simulink model "simple_simulation"  (R2025b)
settings: Solver=ode45  StartTime=0.0  StopTime=30  RelTol=1e-3
values from neighbouring files (symbols this model uses):
  M = SX.zeros(n, n)    [get_wheeled_robot_model.m]    (also in simple_model.m = 19)
  m_w = 1.0    (= 1)    [get_wheeled_robot_model.m]    (also in simple_model.m)
  N = 40    [simple_ocp.m]    (also in solver_ocp.m = 50)
undefined symbols (not defined in the file or in its folder): lx, ly, lz, r, X, Y, Z
libraries: sm_lib x35, nesl_utility x9, simulink x3, slpidlib x1
(part 1 of 2)
settings Model: Creator=oj  LastModifiedBy=itsan
settings SolverCC: AlgebraicLoopSolver=TrustRegion
settings DataIOCC: SaveFormat=StructureWithTime
settings OptimizationCC: LifeSpan=inf
settings DebuggingCC: UnconnectedInputMsg=warning  UnconnectedOutputMsg=warning  UnconnectedLineMsg=warning  SFExecutionAtInitializationDiag=none  ArithmeticOperatorsInVariantConditions=warning
settings HardwareCC: ProdBitPerSizeT=32.0  ProdBitPerPtrDiffT=32.0  ProdWordSize=32.0  ProdHWDeviceType=Specified
settings SFSimCC: CustomCodeUndefinedFunction=UseInterfaceOnly
settings RTWCC: GPUComputeCapability=3.5
settings CodeAppCC: StateflowObjectComments=on

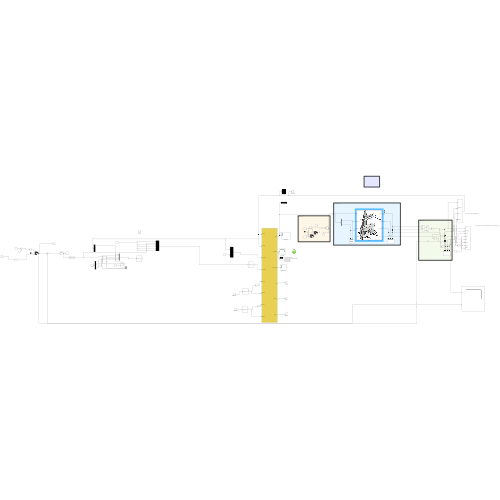
[thumbnail: Simulink's stored preview of the top-level diagram]
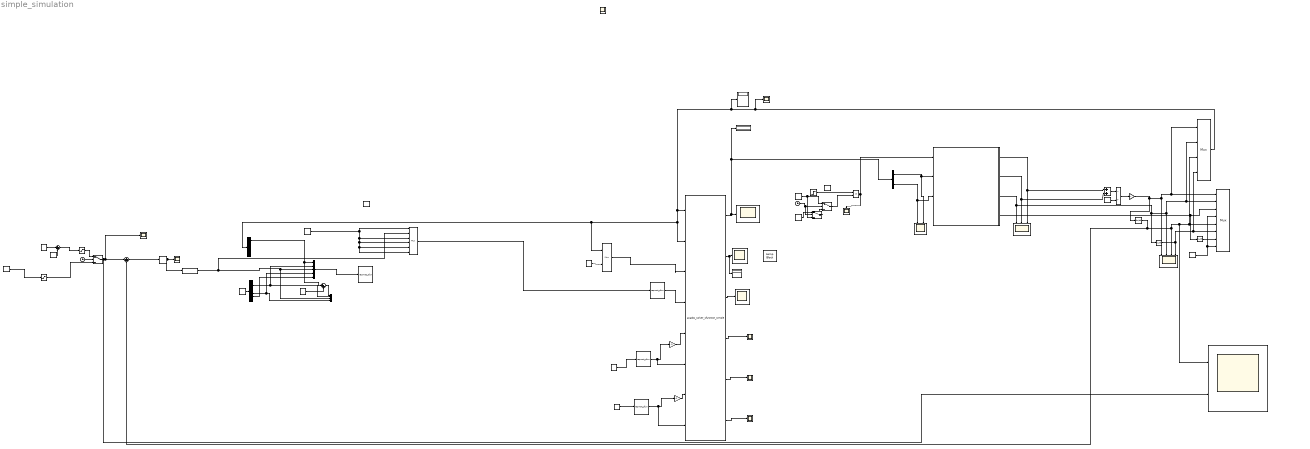
== system simple_simulation ==
  note: [x; beta; x_dot; beta_dot];
  note: 0: successful convergence
      | 1: maximum number of iterations reached
      | 2: line search failed
      | 3: QP solver failed
      | 4: time limit reached
  note: [x; theta_pitch; d_m; theta_a;x_dot; theta_pitch_dot; d_m_dot; theta_a_dot]
  note: Lift control
  note: Simscape model
  note: Calculations
  note: Disturbance
  CPU : Scope
      settings: Description=status  ActiveDisplayYMinimum=-0.000978492283750898  ActiveDisplayYMaximum=0.0013917002145656821  DataLoggingVariableName=ScopeData3
  Clock : Clock
      settings: Decimation=7
  Clock1 : Clock
  Constant : Constant  Value=0
  Constant1 : Constant
  Constant13 : Constant  Value=0
  Constant14 : Constant  Value=2
  Constant15 : Constant
  Constant2 : Constant  Value=[0 0]
  Constant3 : Constant  Value=0
  Constant6 : Constant  Value=2
  Demux : Demux  Outputs=2
  Demux2 : Demux
  Demux3 : Demux  Outputs=6
  Derivative : Derivative
  Derivative1 : Derivative
  Derivative2 : Derivative
  Display : Display
  Display1 : Display
  Divide : Product  Inputs=**
  Divide1 : Product  Inputs=*/
  Gain : Gain  Gain=-1
  Gain1 : Gain  Gain=-1
  Gain2 : Gain  Gain=r
  KKT residual : Scope
      settings: Description=status  ActiveDisplayYMinimum=-0.32883901659053916  ActiveDisplayYMaximum=1.592767698176573  DataLoggingVariableName=ScopeData4
  Lamp : LampBlock  LabelPosition=Hide  DefaultColor=[254.0, 51.0, 10.0]
  Mux : Mux  Inputs=8
      settings: DisplayOption=signals
  Mux1 : Mux
  Mux2 : Mux  Inputs=5
  Mux3 : Mux  Inputs=6
  Mux4 : Mux
      settings: DisplayOption=signals
  Mux5 : Mux  Inputs=2
  OCP status : Scope
      settings: Description=status  ActiveDisplayYMinimum=-2.0851401210050069  ActiveDisplayYMaximum=5.2280116787993132
  PID Controller : slpidlib/PID Controller  Controller=PID  Form=Parallel  TimeDomain=Discrete-time  UseExternalTs=off  SampleTime=-1  IntegratorMethod=Forward Euler  FilterMethod=Forward Euler  ControllerParametersSource=internal  P=2  I=1  UseKiTs=off  D=0  UseExternalDerivativeSource=off  N=100  UseFilter=on  TunerSelectOption=Transfer Function Based (PID Tuner App)  InitialConditionSource=internal  InitialConditionForIntegrator=0  InitialConditionForFilter=0  DifferentiatorICPrevScaledInput=0  ExternalReset=none  TrackingMode=off  Kt=1  LimitOutput=off  SatLimitsSource=internal  UpperSaturationLimit=inf  LowerSaturationLimit=-inf  LinearizeAsGain=on  AntiWindupMode=none  Kb=1  LimitIntegrator=off  UpperIntegratorSaturationLimit=inf  LowerIntegratorSaturationLimit=-inf  POutMin=[]  POutMax=[]  IOutMin=[]  IOutMax=[]  DOutMin=[]  DOutMax=[]  NOutMin=[]  NOutMax=[]  SumOutMin=[]  SumOutMax=[]  SaturationOutMin=[]  SaturationOutMax=[]  PParamMin=[]  PParamMax=[]  IParamMin=[]  IParamMax=[]  DParamMin=[]  DParamMax=[]  NParamMin=[]  NParamMax=[]  KbParamMin=[]  KbParamMax=[]  KtParamMin=[]  KtParamMax=[]  KbOutMin=[]  KbOutMax=[]  KtOutMin=[]  KtOutMax=[]  IntegratorOutMin=[]  IntegratorOutMax=[]  FilterOutMin=[]  FilterOutMax=[]  SumI1OutMin=[]  SumI1OutMax=[]  SumI2OutMin=[]  SumI2OutMax=[]  SumI3OutMin=[]  SumI3OutMax=[]  SumI4OutMin=[]  SumI4OutMax=[]  SumDOutMin=[]  SumDOutMax=[]  DifferentiatorOutMin=[]  DifferentiatorOutMax=[]  FilterDiffOutCoefMin=[]  FilterDiffOutCoefMax=[]  ReciprocalOutMin=[]  ReciprocalOutMax=[]  SumDenOutMin=[]  SumDenOutMax=[]  SumNumOutMin=[]  SumNumOutMax=[]  DivideOutMin=[]  DivideOutMax=[]  UdiffTsProdOutMin=[]  UdiffTsProdOutMax=[]  NTsProdOutMin=[]  NTsProdOutMax=[]  UintegralTsProdOutMin=[]  UintegralTsProdOutMax=[]  UngainTsProdOutMin=[]  UngainTsProdOutMax=[]  ClampingZeroOutDataTypeStr=Inherit: Inherit via back propagation  ClampingZeroOutMin=[]  ClampingZeroOutMax=[]  FilterDenConstantOutDataTypeStr=Inherit: Inherit via back propagation  FilterDenConstantOutMin=[]  FilterDenConstantOutMax=[]  PCopyOutDataTypeStr=Inherit: Inherit via back propagation  PCopyOutMin=[]  PCopyOutMax=[]  NCopyOutDataTypeStr=Inherit: Inherit via back propagation  NCopyOutMin=[]  NCopyOutMax=[]  IntegratorContinuousStateAttributes=''  IntegratorStateMustResolveToSignalObject=off  IntegratorRTWStateStorageClass=Auto  FilterContinuousStateAttributes=''  FilterStateMustResolveToSignalObject=off  FilterRTWStateStorageClass=Auto  ParallelPVariant=InternalParameters  IdealPVariant=Disabled  IVariant=InternalParameters  DVariant=InternalParameters  IntegratorVariant=Discrete  SatVariant=Disabled  AWVariant=Passthrough  PCopyVariant=Disabled  TRVariant=Disabled  FdbkBlocksVariant=Forward  IdealPFdbkVariant=Disabled  SatFdbkVariant=Disabled  DerivativeFilterVariant=ForwardEulerFilter  NVariant=InternalParameters  NCopyVariant=Disabled  FilterICVariant=InternalICsFilter  IntegratorICVariant=InternalICs  ExternalResetVariant=Disabled  TRSumVariant=Passthrough  SumFdbkVariant=Disabled  SumVariant=Sum_PID  TsampFilterVariant=InternalTs  TsampNgainVariant=Passthrough  TsampIntegralVariant=Disabled_SignalSpec  ExternalSaturationOutDataTypeStr=Inherit: Same as second input  DerivativeSourceVariant=ErrorSignal  PreIntVariant=InternalPreInt
  Plant : Subsystem
      mask Display: image('plant.png');
  Ramp : simulink/Sources/Ramp  slope=4  start=1  InitialOutput=0
  Ramp1 : simulink/Sources/Ramp  slope=1  start=1  InitialOutput=0
  Ramp2 : simulink/Sources/Ramp  slope=1  start=15  InitialOutput=0
  S-Function : S-Function  FunctionName=repmat_sfun  Parameters=N-1  SFunctionDeploymentMode=off  EnableBusSupport=off
  S-Function1 : S-Function  FunctionName=acados_solver_sfunction_simple  SFunctionDeploymentMode=off  EnableBusSupport=off
      mask Display:
      | % from the make_sfun file
      | global sfun_input_names sfun_output_names
      | for i = 1:length(sfun_input_names)
      | 	port_label('input', i, sfun_input_names{i})
      | end
      | for i = 1:length(sfun_output_names)
      | 	port_label('output', i, sfun_output_names{i})
      | end
  S-Function3 : S-Function  FunctionName=repmat_sfun  Parameters=N-1  SFunctionDeploymentMode=off  EnableBusSupport=off
  S-Function5 : S-Function  FunctionName=repmat_sfun  Parameters=N-1  SFunctionDeploymentMode=off  EnableBusSupport=off
  S-Function6 : S-Function  FunctionName=repmat_sfun  Parameters=N  SFunctionDeploymentMode=off  EnableBusSupport=off
  SQP iter : Scope
      settings: Description=status  ActiveDisplayYMinimum=0.875  ActiveDisplayYMaximum=2.125  DataLoggingVariableName=ScopeData5
  Saturation : Saturate  UpperLimit=7  LowerLimit=0
  Saturation1 : Saturate  UpperLimit=2  LowerLimit=0
  Scope control : Scope
      settings: ActiveDisplayYMinimum=-0.940224483697417  ActiveDisplayYMaximum=0.84814292592049234  DataLoggingVariableName=ScopeData6
  Scope state : Scope
      settings: ActiveDisplayYMinimum=-5.1246786227559147  ActiveDisplayYMaximum=5.19040547443582  DataLoggingVariableName=ScopeData7
  Scope1 : Scope  NumInputPorts=4
      settings: ActiveDisplayYMinimum=-2.487475277797643  ActiveDisplayYMaximum=2.7538021848706755  DataLoggingVariableName=ScopeData8
  Scope2 : Scope  NumInputPorts=3
      settings: ActiveDisplayYMinimum=-1  ActiveDisplayYMaximum=1  DataLoggingVariableName=ScopeData9
  Scope3 : Scope  NumInputPorts=2
      settings: ActiveDisplayYMinimum=-119.45336825918621  ActiveDisplayYMaximum=75.0803143326759  DataLoggingVariableName=ScopeData10
  Scope{,4..6} (4 alike) : Scope
      Scope4 settings: ActiveDisplayYMinimum=-6.9744188227806294  ActiveDisplayYMaximum=21.518082250301433  DataLoggingVariableName=ScopeData11
      Scope5 settings: ActiveDisplayYMinimum=-0.33598382002949112  ActiveDisplayYMaximum=2.7666726119275413  DataLoggingVariableName=ScopeData12
      Scope6 settings: ActiveDisplayYMinimum=-5.6517884719332452  ActiveDisplayYMaximum=11.007186799770921  DataLoggingVariableName=ScopeData13
      Scope settings: ActiveDisplayYMinimum=-13.79726  ActiveDisplayYMaximum=10.28583
  Scope7 : Scope  NumInputPorts=2
      settings: ActiveDisplayYMinimum=-0.5039307333892511  ActiveDisplayYMaximum=2.5785437278536216  DataLoggingVariableName=ScopeData19
  Signal Specification : SignalSpecification  OutDataTypeStr=double  Dimensions=1
  Step : Step  After=3  SampleTime=0
  Sum : Sum  Inputs=+|+
  Sum3 : Sum  Inputs=|+-
  Sum4 : Sum  Inputs=|++
  Sum5 : Sum  Inputs=|+-
  Switch : Switch  Criteria=u2 > Threshold  Threshold=9  SaturateOnIntegerOverflow=off  InputSameDT=off
  Switch1 : Switch  Criteria=u2 > Threshold  Threshold=7  SaturateOnIntegerOverflow=off  InputSameDT=off
  Switch2 : Switch  Criteria=u2 > Threshold  Threshold=15  SaturateOnIntegerOverflow=off  InputSameDT=off
  limits_inputs : Constant  Value=[100,5,5,5];
  limits_outputs : Constant  Value=[10,10]
  u : Display
  weights : Constant  Value=repmat([5;3;0;1e-3], 244/4, 1)
  x1 ocp : Scope
      settings: Description=status  ActiveDisplayYMinimum=-2.6422889921421415  ActiveDisplayYMaximum=2.2266101006407979  DataLoggingVariableName=ScopeData2
  y_ref4 : Constant  Value=[0; 0; 0; 0; 0; 0]
  wires:
  S-Function1/5 -> CPU/1
  S-Function1/6 -> SQP iter/1
  S-Function1/3 -> KKT residual/1
  Mux4/1 -> Display1/1, S-Function1/2, Mux5/1, Demux2/1, S-Function1/1, Scope state/1  "x"
  S-Function1/4 -> x1 ocp/1
  S-Function1/2 -> OCP status/1, Display/1
  Clock/1 -> Switch1/2, Switch/2
  Constant/1 -> Switch1/3, Switch/1
  Divide/1 -> Scope5/1, Plant/1(dF)
  Switch/1 -> Divide/2
  S-Function1/1 -> Demux/1, u/1, Scope control/1  "u"
  Switch1/1 -> Switch/3
  Constant1/1 -> Switch1/1
  Mux3/1 -> S-Function3/1
  Plant/1(rw_angle) -> Sum/1, Scope2/3  "rw_angle"
  Plant/2(lw_angle) -> Scope2/2, Sum/2  "lw_angle"
  Plant/3(pitch_angle) -> Scope2/1, Mux4/2, Mux/2, Scope1/2, Derivative1/1  "pitch_angle"
  Sum/1 -> Divide1/1
  Constant6/1 -> Divide1/2
  Divide1/1 -> Gain2/1
  Gain2/1 -> Mux4/1, Mux/1, Scope1/1, Derivative/1  "x"
  Derivative/1 -> Scope7/1, Mux/5, Mux4/3, Scope1/3, Sum3/2  "x_dot"
  Derivative1/1 -> Mux/6, Mux4/4, Scope1/4  "pitch_dot"
  Step/1 -> Divide/1
  Mux2/1 -> S-Function/1
  y_ref4/1 -> Demux3/1
  Demux3/4 -> Mux2/4, Mux1/4
  Demux3/5 -> Mux2/5
  Demux2/1 -> Sum4/1, Mux2/1
  Sum3/1 -> PID Controller/1
  PID Controller/1 -> Signal Specification/1, Scope4/1
  Signal Specification/1 -> Mux3/2, Mux2/3, Mux1/3
  Demux3/2 -> Mux2/2, Mux1/2
  Sum4/1 -> Mux1/1
  Constant15/1 -> Sum4/2
  Clock1/1 -> Switch2/2
  Saturation/1 -> Switch2/1
  Sum5/1 -> Saturation/1
  Switch2/1 -> Scope7/2, Sum3/1, Scope6/1
  Gain1/1 -> S-Function1/5
  Gain/1 -> S-Function1/7
  Mux5/1 -> S-Function1/3
  Plant/4(lift_pos) -> Derivative2/1, Mux/3
  Constant3/1 -> Mux/8, Mux/4
  Derivative2/1 -> Mux/7  "pitch_dot"
  S-Function3/1 -> S-Function1/4
  Constant13/1 -> Mux3/3, Mux3/4, Mux3/5, Mux3/6, Mux3/1
  Demux/1 -> Scope3/2, Plant/2(rwTorque)
  Demux/2 -> Plant/3(lwTorque), Scope3/1
  limits_inputs/1 -> S-Function5/1
  S-Function5/1 -> S-Function1/6, Gain1/1
  limits_outputs/1 -> S-Function6/1
  S-Function6/1 -> S-Function1/8, Gain/1
  Ramp1/1 -> Saturation1/1
  Saturation1/1 -> Switch2/3
  Constant2/1 -> Mux5/2
  Constant14/1 -> Sum5/1
  Ramp2/1 -> Sum5/2
